simulink model "BasicAudio"  (R2022b)
settings: Solver=FixedStepDiscrete  StartTime=0.0  StopTime=0.1  RelTol=1e-3  EnableMultiTasking=on
InitFcn:
  | % Initialize model
  | run([ ModelRootName() 'Init.m' ]);
  | 
  | % load library data
  | GainLibrary_data;
model workspace (MAT data in the model file):
  PreampVolumeTable_Idx = Simulink.Signal
  PreampVolumeTable_Idx.DataType = 'auto'
  PreampVolumeTable_Idx.Dimensions = -1
  PreampVolumeTable_Idx.DimensionsMode = 'auto'
  PreampVolumeTable_Idx.Complexity = 'auto'
  PreampVolumeTable_Idx.SampleTime = -1
  PreampVolumeTable_Idx.SamplingMode = 'auto'
  PreampVolumeTable_Idx.InitialValue = 'uint8([0 255 255 255 255 255])'
  Range = Simulink.Signal
  Range.DataType = 'auto'
  Range.Dimensions = -1
  Range.DimensionsMode = 'auto'
  Range.Complexity = 'auto'
  Range.SampleTime = -1
  Range.SamplingMode = 'auto'
  Table_Idx = Simulink.Signal
  Table_Idx.DataType = 'auto'
  Table_Idx.Dimensions = -1
  Table_Idx.DimensionsMode = 'auto'
  Table_Idx.Complexity = 'auto'
  Table_Idx.SampleTime = -1
  Table_Idx.SamplingMode = 'auto'
values from neighbouring files (symbols this model uses):
  ModelCfg = struct()    [BasicAudioInit.m]
libraries: EdgePorts x2, BasicAudioLib x1, FeaturePath x1, HandyTextFile x1, simulink x1, dspsrcs4 x1
settings Model: Creator=kl13806  LastModifiedBy=ra1043664
settings SolverCC: AlgebraicLoopSolver=TrustRegion
settings DataIOCC: ReturnWorkspaceOutputs=off
settings OptimizationCC: DefaultParameterBehavior=Inlined  DefaultUnderspecifiedDataType=single  EfficientTunableParamExpr=on
settings DebuggingCC: InheritedTsInSrcMsg=none  MultiTaskDSMMsg=none  ParameterPrecisionLossMsg=none  ParameterTunabilityLossMsg=error  UnconnectedInputMsg=warning  UnconnectedOutputMsg=warning  UnconnectedLineMsg=warning  UnknownTsInhSupMsg=none  SFUnexpectedBacktrackingDiag=warning  SFNoUnconditionalDefaultTransitionDiag=warning  SFExecutionAtInitializationDiag=none  SFMachineParentedDataDiag=warning  ArithmeticOperatorsInVariantConditions=warning
settings HardwareCC: ProdBitPerPointer=32  ProdBitPerSizeT=32  ProdBitPerPtrDiffT=32  ProdWordSize=32  ProdHWDeviceType=Intel->x86-32 (Windows32)  TargetBitPerPointer=64  TargetBitPerSizeT=64  TargetBitPerPtrDiffT=64  TargetLongLongMode=on  TargetIntDivRoundTo=Zero  TargetEndianess=LittleEndian  TargetWordSize=64  TargetHWDeviceType=MATLAB Host  ProdEqTarget=off
settings ModelReferenceCC: EnableRefExpFcnMdlSchedulingChecks=on
settings SFSimCC: SimUseLocalCustomCode=off  MATLABDynamicMemAlloc=off  CustomCodeUndefinedFunction=UseInterfaceOnly
settings RTWCC: Description=Embedded Coder (host-based shared library target)  SystemTargetFile=ert_shrlib.tlc  GenCodeOnly=on  TemplateMakefile=ert_default_tmf  GenerateReport=on  RetainRTWFile=on  RTWUseLocalCustomCode=off  Toolchain=MinGW64 | gmake (64-bit Windows)  BuildConfiguration=Faster Runs  IncludeHyperlinkInReport=on  LaunchReport=on  GenerateTraceInfo=on  GenerateTraceReport=on  GenerateTraceReportSl=on  GenerateTraceReportSf=on  GenerateTraceReportEml=on  GenerateCodeMetricsReport=on
settings CodeAppCC: ForceParamTrailComments=on  IgnoreCustomStorageClasses=off  OperatorAnnotations=on  SimulinkDataObjDesc=on  SFDataObjDesc=on  MATLABFcnDesc=on  InsertBlockDesc=on  StateflowObjectComments=on  MATLABSourceComments=on
settings STFCustomTargetCC: TargetLangStandard=C99 (ISO)  ParMdlRefBuildCompliant=on  CompOptLevelCompliant=on  CombineOutputUpdateFcns=on  ERTCustomFileBanners=on  SupportNonFinite=off  SupportContinuousTime=off  SupportNonInlinedSFcns=off  RemoveResetFunc=on  SupportVariableSizeSignals=on  MATLABClassNameForMDSCustomization=Simulink.SoftwareTarget.ERTCustomization  ModelStepFunctionPrototypeControlCompliant=on  UseToolchainInfoCompliant=on  SystemTargetFile=ert_shrlib.tlc
settings ERTTargetCC: TargetLangStandard=C99 (ISO)  MultiwordLength=2048  ConcurrentExecutionCompliant=off  SupportNonFinite=off  SupportVariableSizeSignals=on  CPPClassGenCompliant=off  InlinedParameterPlacement=NonHierarchical  ERTCustomFileTemplate=example_file_process.tlc
settings ConfigComp: CovMetricSettings=dw  CovSaveCumulativeToWorkspaceVar=on  CovSaveSingleToWorkspaceVar=on  CovExternalEMLEnable=off

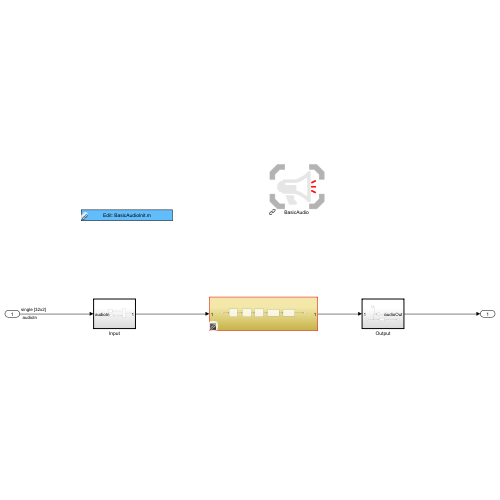
[thumbnail: Simulink's stored preview of the top-level diagram]
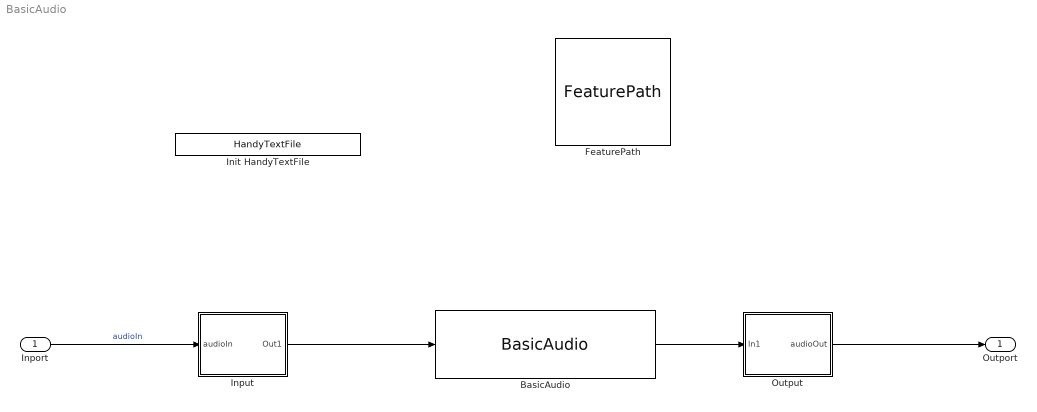
== system BasicAudio ==
  Inport : Inport  OutDataTypeStr=single  PortDimensions=[ModelCfg.In.FrameSamples ModelCfg.In.ChannelCount]  SampleTime=1/ModelCfg.In.SampleRateInHertz * ModelCfg.In.FrameSamples
  BasicAudio : BasicAudioLib/BasicAudio  SystemSampleTime=-1  VariantActivationTime=update diagram  Latency=0  AutoFrameSizeCalculation=off
  FeaturePath : FeaturePath/FeaturePath  FeatureName=BasicAudio  IsGroup=on  GroupNumber=-1  IsModule=off  TriggerInit=[45 -501 160 -394]
      settings: SourceProductName=Bose Talaria
  Init HandyTextFile : HandyTextFile/HandyTextFile  TemplateSource=<dialog fields>  FileSuffix=Init.m  OpenDialogOnLoad=off  UseThisBlockName=off  AddGrandParentNamePrefix=off  TheDefaultText=|  ShowInLibBrowser=on
      | % Setup model parameters for each "Init" callback (e.g. update diagram)
      | sample_rate_in_hertz = 44100;
      | frame_size = 32;
      | sysin_channel_count = 2;
      | 
      | % setup simulation RTC data
      | run([ModelRootName() 'SimEvents.m']);
      settings: SourceProductName=Bose Talaria
  Input : Subsystem  TreatAsAtomicUnit=on
  Output : Subsystem  TreatAsAtomicUnit=on
  Outport : Outport  VectorParamsAs1DForOutWhenUnconnected=off
  wires:
  Inport/1 -> Input/1(audioIn)  "audioIn"
  Input/1(Out1) -> BasicAudio/1
  BasicAudio/1 -> Output/1(In1)
  Output/1(audioOut) -> Outport/1

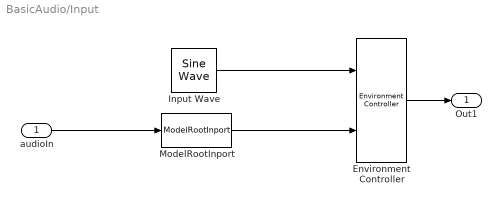
== system BasicAudio/Input ==
  audioIn : Inport
  Environment Controller : simulink/Signal Routing/Environment Controller
  Input Wave : dspsrcs4/Sine Wave  Amplitude=1  Frequency=500*(1:ModelCfg.In.ChannelCount)  Phase=0  SampleMode=Discrete  OutComplex=Real  CompMethod=Trigonometric fcn  TableSize=Speed  SampleTime=1/ModelCfg.In.SampleRateInHertz  SamplesPerFrame=ModelCfg.In.FrameSamples  ResetState=Restart at time zero  OutputFrames=off  dataType=single  wordLen=16  udDataType=sfix(16)  fracBitsMode=Best precision  numFracBits=15  OutDataTypeStr=single  LastOutDataTypeStr=single
  ModelRootInport : EdgePorts/ModelRootInport  Config=ModelCfg.In
      settings: SourceProductName=Bose Talaria
  Out1 : Outport
  wires:
  ModelRootInport/1 -> Environment Controller/2
  Input Wave/1 -> Environment Controller/1
  Environment Controller/1 -> Out1/1
  audioIn/1 -> ModelRootInport/1

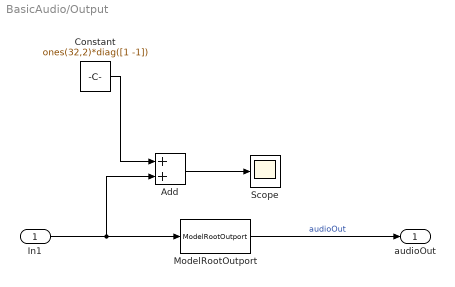
== system BasicAudio/Output ==
  In1 : Inport
  Add : Sum
  Constant : Constant  Value=ones(32,2)*diag([1 -1])
  ModelRootOutport : EdgePorts/ModelRootOutport  Config=ModelCfg.Out
      settings: SourceProductName=Bose Talaria
  Scope : Scope
  audioOut : Outport
  wires:
  In1/1 -> ModelRootOutport/1, Add/2
  Add/1 -> Scope/1
  Constant/1 -> Add/1
  ModelRootOutport/1 -> audioOut/1  "audioOut"
